simulink model "irep_force_control_simu"  (Simulink 8.5)
settings: Solver=ode3  StartTime=0.0  StopTime=inf  FixedStep=dt  RelTol=1e-3
InitFcn:
  | IREP_DEPENDENCY
  | init_omni
  | init_filters
  | init_invivo
  | init_telemanipulation
  | init_parker_xyz
  | init_magnetic_tracker
  | init_loadcell
  | init_scopes
  | init_homing
  | init_force_control
  | init_xpc_invivo_simu
undefined symbols (not defined in the file): ang_vel_scale, B_simu, beta, camera_home_voltage, counter_offset, dt, dt_trakstar, E_Y, encoder_counts, epsilon_robust_inverse, gear_ratio, HomingFineEps, HomingRoughEps, HomingRoughVelocity, I1_primary, I1_secondary, I2_primary, I2_secondary, irep_parameters_left, irep_parameters_right, joystick_filter_coeffs, K_d, K_i, K_naive_inv, K_p, k_right, L1l, L1r, L2l, L2r, L_zeus, left_arm_home_voltage, left_x0_parallelogram, LeftArmHomingDirectionVector, LeftArmHomingIntGain, lin_vel_scale, LOADCELL_BIAS, LOADCELL_GAIN, max_conf_space_speed, N_joystick, N_pots, N_trakstar, OmegaMax, OmegaMin, orientation_epsilon, position_epsilon, pots_filter_coeffs, q_eps_backlash, quadrature_mode, r, right_arm_home_voltage, RightArmHomingDirectionVector, RightArmHomingIntGain, screw_pitch, statics_param, tau_compression_bias, tau_compression_gains, tau_neutral_deadband, tau_tension_bias, tau_tension_gains ... (+14)
libraries: slrtlib x38, xpcrtudplib x13, xpcobsoletelib x13, simulink x6, dspswit3 x2, dspsigops x1
(part 1 of 6)
settings Model: Creator=Andrea  LastModifiedBy=Long
settings SolverCC: EnableConcurrentExecution=on
settings OptimizationCC: BlockReduction=off  OptimizeBlockIOStorage=off  BufferReuse=off  GlobalBufferReuse=off  ExpressionFolding=off  LocalBlockOutputs=off  OptimizeModelRefInitCode=on
settings DebuggingCC: SolverPrmCheckMsg=warning  MultiTaskCondExecSysMsg=warning  MultiTaskRateTransMsg=warning  FcnCallInpInsideContextMsg=UseLocalSettings
settings HardwareCC: ProdIntDivRoundTo=Zero  ProdEndianess=LittleEndian  ProdLongLongMode=on  ProdHWDeviceType=Generic->32-bit x86 compatible
settings SFSimCC: SimParseCustomCode=off
settings RTWCC: SystemTargetFile=slrtert.tlc  TemplateMakefile=slrtert_default_tmf  Description=Simulink Real-Time (ERT)  RTWCompilerOptimization=on
settings CodeAppCC: CustomSymbolStrType=$N$R$M  InternalIdentifier=Classic
settings SimulinkRealTimeERTCC: TargetFcnLib=ansi_tfl_table_tmw.mat  GenFloatMathFcnCalls=NOT IN USE  TargetLangStandard=C89/C90 (ANSI)  CodeReplacementLibrary=XPC_BLAS  UtilityFuncGeneration=Auto  ERTMultiwordTypeDef=System defined  ERTMultiwordLength=256  MultiwordLength=2048  GenerateFullHeader=on  InferredTypesCompatibility=off  GenerateSampleERTMain=off  GenerateTestInterfaces=off  ModelReferenceCompliant=on  ParMdlRefBuildCompliant=on  CompOptLevelCompliant=on  ConcurrentExecutionCompliant=on  IncludeMdlTerminateFcn=on  GeneratePreprocessorConditionals=Disable all  CombineOutputUpdateFcns=off  CombineSignalStateStructs=off  SuppressErrorStatus=off  ERTFirstTimeCompliant=off  IncludeFileDelimiter=Auto  ERTCustomFileBanners=off  SupportAbsoluteTime=on  LogVarNameModifier=rt_  MatFileLogging=on  MultiInstanceERTCode=off  CodeInterfacePackaging=Nonreusable function  SupportNonFinite=on  SupportComplex=on  PurelyIntegerCode=off  SupportContinuousTime=on  SupportNonInlinedSFcns=on  SupportVariableSizeSignals=off  ParenthesesLevel=Nominal  CastingMode=Nominal  MATLABClassNameForMDSCustomization=xpcAperiodicCustomization  ModelStepFunctionPrototypeControlCompliant=off  CPPClassGenCompliant=off  AutosarCompliant=off  GRTInterface=on  GenerateAllocFcn=off  GenerateSharedConstants=on  GenerateASAP2=off  ExtModeTransport=0  ExtModeStaticAlloc=off  ExtModeStaticAllocSize=1000000  ExtModeTesting=off  InlinedParameterPlacement=NonHierarchical  TargetOS=BareBoardExample  MultiInstanceErrorCode=Error  RateGroupingCode=on  RootIOFormat=Individual arguments  RTWCAPIRootIO=off  EnableDataOwnership=off  ERTFilePackagingFormat=Modular  PreserveExpressionOrder=off  PreserveIfCondition=off  ConvertIfToSwitch=off  PreserveExternInFcnDecls=on  SuppressUnreachableDefaultCases=off  EnableSignedLeftShifts=on  IndentStyle=K&R  IndentSize=2  EnableUserReplacementTypes=off  MaxIdInt32=MAX_int32_T  MinIdInt32=MIN_int32_T  MaxIdUint32=MAX_uint32_T  MaxIdInt16=MAX_int16_T  MinIdInt16=MIN_int16_T  MaxIdUint16=MAX_uint16_T  MaxIdInt8=MAX_int8_T  MinIdInt8=MIN_int8_T  MaxIdUint8=MAX_uint8_T  BooleanTrueId=true  BooleanFalseId=false  MemSecPackage=--- None ---  MemSecDataConstants=Default  MemSecDataIO=Default  MemSecDataInternal=Default  MemSecDataParameters=Default  MemSecFuncInitTerm=Default  MemSecFuncExecute=Default  MemSecFuncSharedUtil=Default  GlobalDataDefinition=Auto  GlobalDataReference=Auto  ERTSrcFileBannerTemplate=ert_code_template.cgt  ERTHdrFileBannerTemplate=ert_code_template.cgt  ERTDataSrcFileTemplate=ert_code_template.cgt  ERTDataHdrFileTemplate=ert_code_template.cgt  ERTCustomFileTemplate=example_file_process.tlc  SignalDisplayLevel=10  ParamTuneLevel=10  InitialValueSource=Model  RTWCAPISignals=off  RTWCAPIParams=on  RTWCAPIStates=off  RL32ModeModifier=Real-Time  ExtMode=on  ExtModeMexFile=ext_xpc  ExtModeIntrfLevel=Level2 - Open  ExtModeArmWhenConnect=off  RL32LogTETModifier=on  RL32LogBufSizeModifier=100000  xPCTaskExecutionProfile=off  xPCRL32EventNumber=5000  RL32IRQSourceModifier=Timer  xPCIRQSourceBoard=None/Other  xPCIOIRQSlot=-1  xpcObjCom=off  xPCGenerateASAP2=off  xPCGenerateXML=off  RL32ObjectName=tg  xPCisDownloadable=off  xPCisDefaultEnv=on  xPCisModelTimeout=on  xPCModelTimeoutSecs=5  xpcDblBuff=off  xPCLoadParamSetFile=off  xPCConcurrentTasks=off  xPCEnableSFAnimation=off

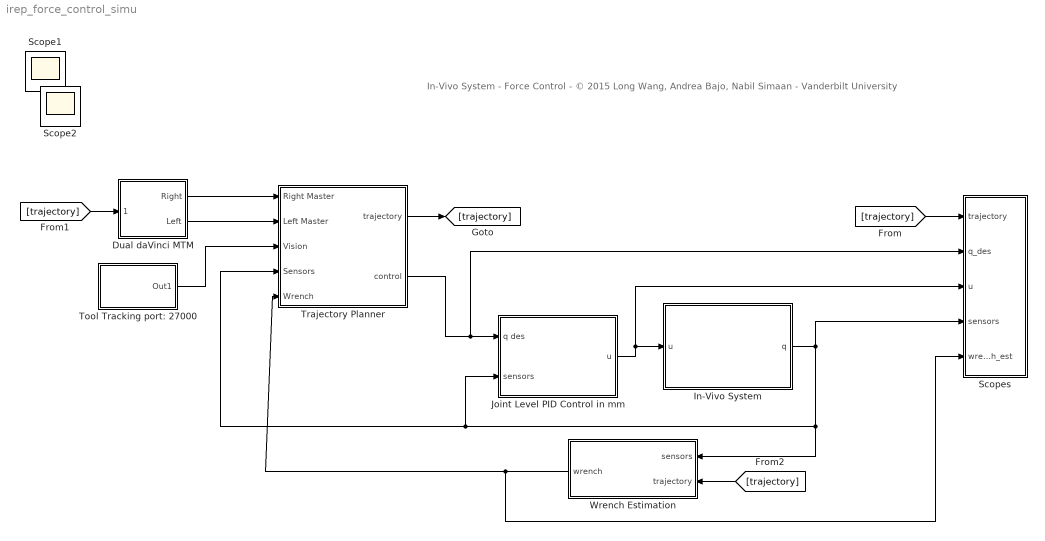
== system irep_force_control_simu ==
  note: In-Vivo System - Force Control - © 2015 Long Wang, Andrea Bajo, Nabil Simaan - Vanderbilt University
  Dual daVinci MTM : Subsystem
      mask Display: image(imread('davinci_doc.jpg'));
  In-Vivo System : Subsystem
      mask Display: image(imread('irep.png'));
  Joint Level PID Control in mm : Subsystem
  Scopes : Subsystem
  Tool Tracking port: 27000 : Subsystem  TreatAsAtomicUnit=on
  Trajectory Planner : Subsystem
  Wrench Estimation : Subsystem
  Scope1 : Scope
      settings: MaxDataPoints=7500
  Scope2 : Scope
      settings: MaxDataPoints=7500
  wires:
  In-Vivo System/1(q) -> Scopes/4(sensors), Trajectory Planner/4(Sensors), Joint Level PID Control in mm/2(sensors), Wrench Estimation/1(sensors)
  Trajectory Planner/2(control) -> Joint Level PID Control in mm/1(q des), Scopes/2(q_des)
  Tool Tracking port: 27000/1(Out1) -> Trajectory Planner/3(Vision)
  Dual daVinci MTM/2(Left) -> Trajectory Planner/2(Left Master)
  Dual daVinci MTM/1(Right) -> Trajectory Planner/1(Right Master)
  Wrench Estimation/1(wrench) -> Scopes/5(wrench_est), Trajectory Planner/5(Wrench)
  Trajectory Planner/1(trajectory) -> [trajectory]
  [trajectory] -> Scopes/1(trajectory)
  [trajectory] -> Dual daVinci MTM/1(trajectory)
  [trajectory] -> Wrench Estimation/2(trajectory)
  Joint Level PID Control in mm/1(u) -> Scopes/3(u), In-Vivo System/1(u)

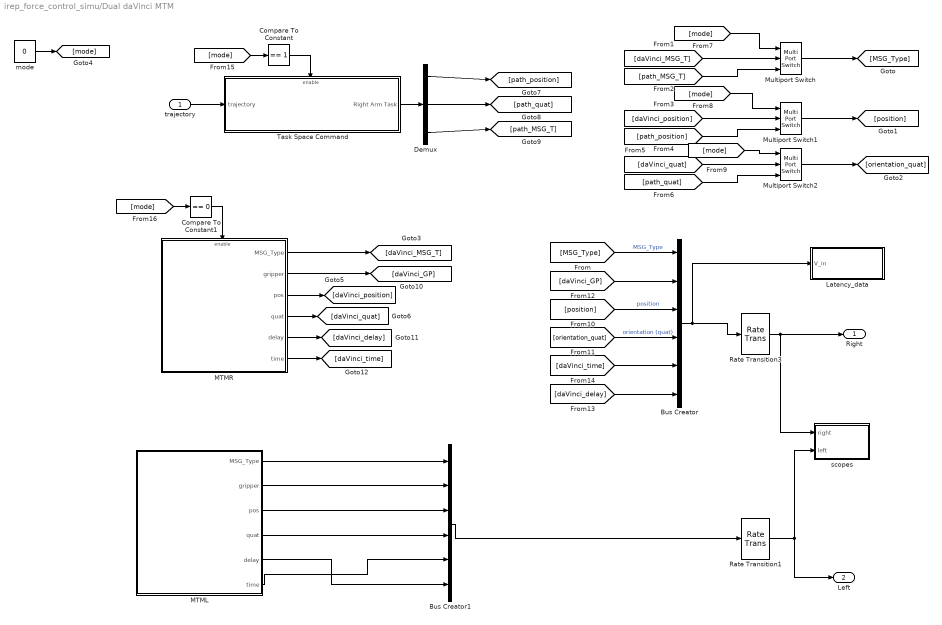
== system irep_force_control_simu/Dual daVinci MTM ==
  trajectory : Inport
  Bus Creator : BusCreator  Inputs=6
  Bus Creator1 : BusCreator  Inputs=6
  Compare To Constant : simulink/Logic and Bit Operations/Compare To Constant  relop===  const=1  OutDataTypeStr=boolean
  Compare To Constant1 : simulink/Logic and Bit Operations/Compare To Constant  relop===  const=0  OutDataTypeStr=boolean
  Demux : Demux  Outputs=[3,4,1]
  Latency_data : Subsystem
  MTML : Subsystem
  MTMR : Subsystem
  Multiport Switch : MultiPortSwitch  DataPortOrder=Zero-based contiguous  Inputs=2  zeroidx=on
  Multiport Switch1 : MultiPortSwitch  DataPortOrder=Zero-based contiguous  Inputs=2  zeroidx=on
  Multiport Switch2 : MultiPortSwitch  DataPortOrder=Zero-based contiguous  Inputs=2  zeroidx=on
  Rate Transition1 : RateTransition  OutPortSampleTime=dt
  Rate Transition3 : RateTransition  OutPortSampleTime=dt
  Task Space Command : Subsystem  TreatAsAtomicUnit=on
  mode : Constant  Value=0
  scopes : Subsystem
  Right : Outport
  Left : Outport  Port=2
  wires:
  Bus Creator/1 -> Latency_data/1(V_in), Rate Transition3/1
  Bus Creator1/1 -> Rate Transition1/1
  Rate Transition3/1 -> Right/1, scopes/1(right)
  Rate Transition1/1 -> Left/1, scopes/2(left)
  Multiport Switch/1 -> [MSG_Type]
  [MSG_Type] -> Bus Creator/1  "MSG_Type"
  Multiport Switch1/1 -> [position]
  Multiport Switch2/1 -> [orientation_quat]
  [daVinci_MSG_T] -> Multiport Switch/2
  [path_MSG_T] -> Multiport Switch/3
  [daVinci_position] -> Multiport Switch1/2
  [path_position] -> Multiport Switch1/3
  [daVinci_quat] -> Multiport Switch2/2
  [path_quat] -> Multiport Switch2/3
  mode/1 -> [mode]
  [mode] -> Multiport Switch/1
  [mode] -> Multiport Switch1/1
  [mode] -> Multiport Switch2/1
  [position] -> Bus Creator/3  "position"
  [orientation_quat] -> Bus Creator/4  "orientation (quat)"
  trajectory/1 -> Task Space Command/1(trajectory)
  Task Space Command/1(Right Arm Task) -> Demux/1
  MTMR/4(quat) -> [daVinci_quat]
  MTMR/3(pos) -> [daVinci_position]
  MTMR/1(MSG_Type) -> [daVinci_MSG_T]
  MTMR/2(gripper) -> [daVinci_GP]
  [daVinci_GP] -> Bus Creator/2
  MTMR/5(delay) -> [daVinci_delay]
  [daVinci_delay] -> Bus Creator/6
  MTMR/6(time) -> [daVinci_time]
  [daVinci_time] -> Bus Creator/5
  [mode] -> Compare To Constant/1
  Compare To Constant/1 -> Task Space Command/Enable
  [mode] -> Compare To Constant1/1
  Compare To Constant1/1 -> MTMR/Enable
  MTML/1(MSG_Type) -> Bus Creator1/1
  MTML/2(gripper) -> Bus Creator1/2
  MTML/3(pos) -> Bus Creator1/3
  MTML/4(quat) -> Bus Creator1/4
  MTML/6(time) -> Bus Creator1/5
  MTML/5(delay) -> Bus Creator1/6
  Demux/1 -> [path_position]
  Demux/2 -> [path_quat]
  Demux/3 -> [path_MSG_T]

== system irep_force_control_simu/In-Vivo System ==
  u : Inport
  ATI FT Sensor : Subsystem
  Bus Creator : BusCreator  Inputs=7
  CONTEC CARDS : Subsystem
  Count to mm : Subsystem
  D/A : Subsystem
  Digital_Inputs : Subsystem
  Loadcells : Subsystem
  Magnetic Tracker 125 Hz : Subsystem  TreatAsAtomicUnit=on
      mask Display: %image(imread('trakSTAR.jpg'));
  Motor Enable : Subsystem
  Potentiometers : Subsystem
  Terminator : Terminator
  motor simulation : Subsystem
  q : Outport
  wires:
  CONTEC CARDS/1(Out1) -> Count to mm/1(counts)
  u/1 -> D/A/1(In1), motor simulation/1(u)
  Potentiometers/1(Pots) -> Bus Creator/2  "A/D signals"
  Bus Creator/1 -> q/1
  Digital_Inputs/1(foot switches) -> Bus Creator/3  "foot switches"
  Digital_Inputs/2(Pot_connect) -> Bus Creator/4  "Pots_Connect"
  ATI FT Sensor/1(Forces) -> Bus Creator/6  "ATI"
  Loadcells/1(loadcell) -> Bus Creator/7  "force_sensing"
  Magnetic Tracker 125 Hz/1(TrakStar) -> Bus Creator/5  "Magnetic Sensors"
  motor simulation/1(q_cur_system) -> Bus Creator/1  "q"
  Count to mm/1(q_cur_system) -> Terminator/1  "q"

== system irep_force_control_simu/Joint Level PID Control in mm ==
  q des : Inport
  sensors : Inport  Port=2
  Bus Creator : Subsystem
  Bus selector : Subsystem
  Enable Control : Constant  Value=0
  PID Compensator : Subsystem
  Sum : Sum  Inputs=|+-  SampleTime=dt
  u : Outport
  wires:
  q des/1 -> Sum/1
  Sum/1 -> PID Compensator/1(e)
  sensors/1 -> Bus selector/1(sensors)
  Bus selector/1(Out1) -> Sum/2
  PID Compensator/1(u) -> Bus Creator/1(In1)
  Bus Creator/1(Out1) -> u/1
  Enable Control/1 -> PID Compensator/Enable

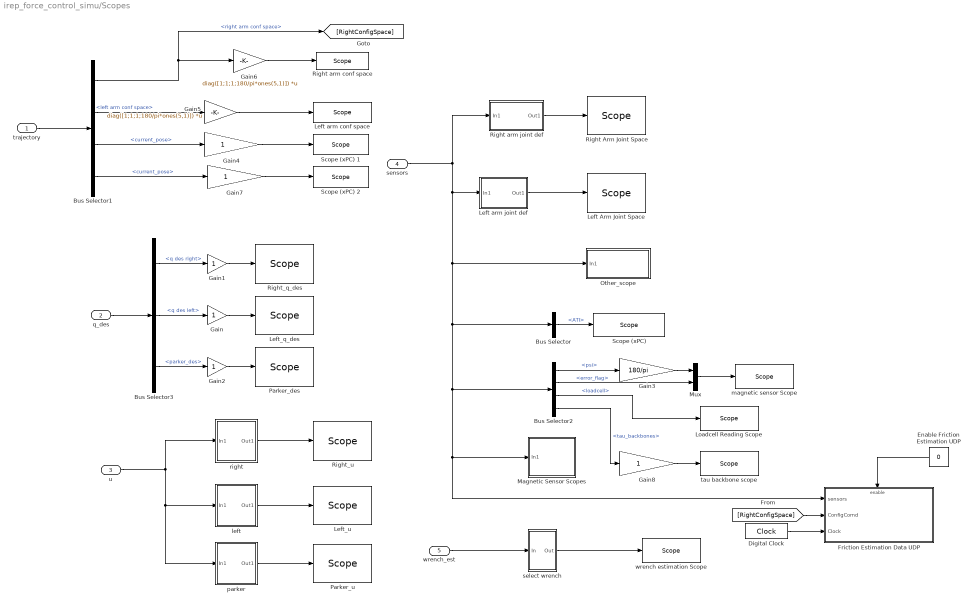
== system irep_force_control_simu/Scopes ==
  trajectory : Inport
  q_des : Inport  Port=2
  u : Inport  Port=3
  sensors : Inport  Port=4
  wrench_est : Inport  Port=5
  Bus Selector : BusSelector  OutputSignals=ATI
  Bus Selector1 : BusSelector  OutputSignals=right arm.right arm conf space,left arm.left arm conf space,right arm.current_pose,left arm.current_pose
  Bus Selector2 : BusSelector  OutputSignals=Magnetic Sensors.psi,Magnetic Sensors.error_flag,force_sensing.loadcell,force_sensing.tau_backbones
  Bus Selector3 : BusSelector  OutputSignals=q des right,q des left,parker_des
  Digital Clock : DigitalClock  SampleTime=dt
  Enable Friction Estimation UDP : Constant  Value=0
  Friction Estimation Data UDP : Subsystem
  Gain{,1..2,4,7..8} (6 alike) : Gain
  Gain3 : Gain  Gain=180/pi
  Gain5 : Gain  Gain=diag([1;1;1;180/pi*ones(5,1)])  Multiplication=Matrix(K*u)
  Gain6 : Gain  Gain=diag([1;1;1;180/pi*ones(5,1)])  Multiplication=Matrix(K*u)
  Left Arm Joint Space : slrtlib/Displays and Logging/Scope   scopeno=5  scopetype=Host  autostart=on  viewmode=Numerical  formatstr=scope_format_left_joint_space  grid=on  ylimits=[0,0]  nosamples=10  noprepostsamples=0  interleave=1  triggermode=FreeRun  triggersignal=1  trigsignalfromport=off  triggerlevel=0.0  triggerslope=Either  triggerscope=1  triggersample=0  filename=weights1.dat  mode=Lazy  writesize=512  autorestart=off  dynamicfilemode=off  maxwritefilesize=512*1024^2
  Left arm conf space : slrtlib/Displays and Logging/Scope   scopeno=10  scopetype=Target  autostart=on  viewmode=Numerical  formatstr=scope_format_left_config_space  grid=on  ylimits=[0,0]  nosamples=10  noprepostsamples=0  interleave=1  triggermode=FreeRun  triggersignal=1  trigsignalfromport=off  triggerlevel=0.0  triggerslope=Either  triggerscope=1  triggersample=0  filename=weights.dat  mode=Lazy  writesize=512  autorestart=off  dynamicfilemode=off  maxwritefilesize=512*1024^2
  Left arm joint def : Subsystem
  Left_q_des : slrtlib/Displays and Logging/Scope   scopeno=13  scopetype=Target  autostart=on  viewmode=Numerical  formatstr=scope_format_left_q_des  grid=on  ylimits=[0,0]  nosamples=10  noprepostsamples=0  interleave=1  triggermode=FreeRun  triggersignal=1  trigsignalfromport=off  triggerlevel=0.0  triggerslope=Either  triggerscope=1  triggersample=0  filename=weights.dat  mode=Lazy  writesize=512  autorestart=off  dynamicfilemode=off  maxwritefilesize=512*1024^2
  Left_u : slrtlib/Displays and Logging/Scope   scopeno=15  scopetype=Host  autostart=on  viewmode=Numerical  formatstr=scope_format_left_u  grid=on  ylimits=[0,0]  nosamples=10  noprepostsamples=0  interleave=1  triggermode=FreeRun  triggersignal=1  trigsignalfromport=off  triggerlevel=0.0  triggerslope=Either  triggerscope=1  triggersample=0  filename=weights.dat  mode=Lazy  writesize=512  autorestart=off  dynamicfilemode=off  maxwritefilesize=512*1024^2
  Loadcell Reading Scope : slrtlib/Displays and Logging/Scope   scopeno=29  scopetype=Host  autostart=on  viewmode=Numerical  formatstr=scope_format_Loadcell  grid=on  ylimits=[0,0]  nosamples=25  noprepostsamples=0  interleave=1  triggermode=FreeRun  triggersignal=1  trigsignalfromport=off  triggerlevel=0.0  triggerslope=Either  triggerscope=1  triggersample=0  filename=data.dat  mode=Lazy  writesize=512  autorestart=off  dynamicfilemode=off  maxwritefilesize=512*1024^2
  Magnetic Sensor Scopes : Subsystem
  Mux : Mux  Inputs=2
  Other_scope : Subsystem
  Parker_des : slrtlib/Displays and Logging/Scope   scopeno=17  scopetype=Host  autostart=on  viewmode=Numerical  formatstr=scope_format_parker_des  grid=on  ylimits=[0,0]  nosamples=10  noprepostsamples=0  interleave=1  triggermode=FreeRun  triggersignal=1  trigsignalfromport=off  triggerlevel=0.0  triggerslope=Either  triggerscope=1  triggersample=0  filename=weights.dat  mode=Lazy  writesize=512  autorestart=off  dynamicfilemode=off  maxwritefilesize=512*1024^2
  Parker_u : slrtlib/Displays and Logging/Scope   scopeno=16  scopetype=Host  autostart=on  viewmode=Numerical  formatstr=scope_format_parker_u  grid=on  ylimits=[0,0]  nosamples=10  noprepostsamples=0  interleave=1  triggermode=FreeRun  triggersignal=1  trigsignalfromport=off  triggerlevel=0.0  triggerslope=Either  triggerscope=1  triggersample=0  filename=weights.dat  mode=Lazy  writesize=512  autorestart=off  dynamicfilemode=off  maxwritefilesize=512*1024^2
  Right Arm Joint Space : slrtlib/Displays and Logging/Scope   scopeno=3  scopetype=Host  autostart=on  viewmode=Numerical  formatstr=scope_format_right_joint_space  grid=on  ylimits=[0,0]  nosamples=10  noprepostsamples=0  interleave=1  triggermode=FreeRun  triggersignal=1  trigsignalfromport=off  triggerlevel=0.0  triggerslope=Either  triggerscope=1  triggersample=0  filename=weights1.dat  mode=Lazy  writesize=512  autorestart=off  dynamicfilemode=off  maxwritefilesize=512*1024^2
  Right arm conf space : slrtlib/Displays and Logging/Scope   scopeno=9  scopetype=Host  autostart=on  viewmode=Numerical  formatstr=scope_format_right_config_space  grid=on  ylimits=[0,0]  nosamples=10  noprepostsamples=0  interleave=1  triggermode=FreeRun  triggersignal=1  trigsignalfromport=off  triggerlevel=0.0  triggerslope=Either  triggerscope=1  triggersample=0  filename=weights.dat  mode=Lazy  writesize=512  autorestart=off  dynamicfilemode=off  maxwritefilesize=512*1024^2
  Right arm joint def : Subsystem
  Right_q_des : slrtlib/Displays and Logging/Scope   scopeno=12  scopetype=Host  autostart=on  viewmode=Numerical  formatstr=scope_format_right_q_des  grid=on  ylimits=[0,0]  nosamples=10  noprepostsamples=0  interleave=1  triggermode=FreeRun  triggersignal=1  trigsignalfromport=off  triggerlevel=0.0  triggerslope=Either  triggerscope=1  triggersample=0  filename=weights.dat  mode=Lazy  writesize=512  autorestart=off  dynamicfilemode=off  maxwritefilesize=512*1024^2
  Right_u : slrtlib/Displays and Logging/Scope   scopeno=14  scopetype=Host  autostart=on  viewmode=Numerical  formatstr=scope_format_right_config_space  grid=on  ylimits=[0,0]  nosamples=10  noprepostsamples=0  interleave=1  triggermode=FreeRun  triggersignal=1  trigsignalfromport=off  triggerlevel=0.0  triggerslope=Either  triggerscope=1  triggersample=0  filename=weights.dat  mode=Lazy  writesize=512  autorestart=off  dynamicfilemode=off  maxwritefilesize=512*1024^2
  "Scope (xPC) " : slrtlib/Displays and Logging/Scope   scopeno=20  scopetype=Host  autostart=on  viewmode=Numerical  formatstr=scope_format_ATI_wrench  grid=on  ylimits=[0,0]  nosamples=25  noprepostsamples=0  interleave=1  triggermode=FreeRun  triggersignal=1  trigsignalfromport=off  triggerlevel=0.0  triggerslope=Either  triggerscope=1  triggersample=0  filename=data.dat  mode=Lazy  writesize=512  autorestart=off  dynamicfilemode=off  maxwritefilesize=512*1024^2
  Scope (xPC) 1 : slrtlib/Displays and Logging/Scope   scopeno=36  scopetype=Host  autostart=on  viewmode=Numerical  formatstr=scope_format_right_task_space_cur  grid=on  ylimits=[0,0]  nosamples=25  noprepostsamples=0  interleave=1  triggermode=FreeRun  triggersignal=1  trigsignalfromport=off  triggerlevel=0.0  triggerslope=Either  triggerscope=1  triggersample=0  filename=data.dat  mode=Lazy  writesize=512  autorestart=off  dynamicfilemode=off  maxwritefilesize=512*1024^2
  Scope (xPC) 2 : slrtlib/Displays and Logging/Scope   scopeno=37  scopetype=Host  autostart=on  viewmode=Numerical  formatstr=scope_format_left_task_space_cur  grid=on  ylimits=[0,0]  nosamples=25  noprepostsamples=0  interleave=1  triggermode=FreeRun  triggersignal=1  trigsignalfromport=off  triggerlevel=0.0  triggerslope=Either  triggerscope=1  triggersample=0  filename=data.dat  mode=Lazy  writesize=512  autorestart=off  dynamicfilemode=off  maxwritefilesize=512*1024^2
  left : Subsystem
  magnetic sensor Scope : slrtlib/Displays and Logging/Scope   scopeno=33  scopetype=Host  autostart=on  viewmode=Numerical  formatstr=scope_format_megnetic_psi  grid=on  ylimits=[0,0]  nosamples=25  noprepostsamples=0  interleave=1  triggermode=FreeRun  triggersignal=1  trigsignalfromport=off  triggerlevel=0.0  triggerslope=Either  triggerscope=1  triggersample=0  filename=data.dat  mode=Lazy  writesize=512  autorestart=off  dynamicfilemode=off  maxwritefilesize=512*1024^2
  parker : Subsystem
  right : Subsystem
  select wrench : Subsystem
  tau backbone scope : slrtlib/Displays and Logging/Scope   scopeno=34  scopetype=Host  autostart=on  viewmode=Numerical  formatstr=scope_format_tau_backbones  grid=on  ylimits=[0,0]  nosamples=50  noprepostsamples=0  interleave=1  triggermode=FreeRun  triggersignal=1  trigsignalfromport=off  triggerlevel=0.0  triggerslope=Either  triggerscope=1  triggersample=0  filename=data.dat  mode=Lazy  writesize=512  autorestart=off  dynamicfilemode=off  maxwritefilesize=512*1024^2
  wrench estimation Scope : slrtlib/Displays and Logging/Scope   scopeno=35  scopetype=Host  autostart=on  viewmode=Numerical  formatstr=scope_format_wrench_est_right_arm  grid=on  ylimits=[0,0]  nosamples=25  noprepostsamples=0  interleave=1  triggermode=FreeRun  triggersignal=1  trigsignalfromport=off  triggerlevel=0.0  triggerslope=Either  triggerscope=1  triggersample=0  filename=data.dat  mode=Lazy  writesize=512  autorestart=off  dynamicfilemode=off  maxwritefilesize=512*1024^2
  wires:
  sensors/1 -> Other_scope/1(In1), Bus Selector/1, Bus Selector2/1, Magnetic Sensor Scopes/1(In1), Friction Estimation Data UDP/1(sensors), Left arm joint def/1(In1), Right arm joint def/1(In1)
  trajectory/1 -> Bus Selector1/1
  Bus Selector1/1 -> [RightConfigSpace], Gain6/1  "<right arm conf space>"
  Bus Selector1/2 -> Gain5/1  "<left arm conf space>"
  q_des/1 -> Bus Selector3/1
  Bus Selector3/1 -> Gain1/1  "<q des right>"
  Bus Selector3/2 -> Gain/1  "<q des left>"
  u/1 -> right/1(In1), left/1(In1), parker/1(In1)
  right/1(Out1) -> Right_u/1
  left/1(Out1) -> Left_u/1
  Gain/1 -> Left_q_des/1
  Gain1/1 -> Right_q_des/1
  parker/1(Out1) -> Parker_u/1
  Bus Selector3/3 -> Gain2/1  "<parker_des>"
  Gain2/1 -> Parker_des/1
  Right arm joint def/1(Out1) -> Right Arm Joint Space/1
  Left arm joint def/1(Out1) -> Left Arm Joint Space/1
  Bus Selector/1 -> "Scope (xPC) "/1  "<ATI>"
  Bus Selector2/1 -> Gain3/1  "<psi>"
  [RightConfigSpace] -> Friction Estimation Data UDP/2(ConfigComd)
  Enable Friction Estimation UDP/1 -> Friction Estimation Data UDP/Enable
  Digital Clock/1 -> Friction Estimation Data UDP/3(Clock)
  Bus Selector2/3 -> Loadcell Reading Scope/1  "<loadcell>"
  Bus Selector2/4 -> Gain8/1  "<tau_backbones>"
  wrench_est/1 -> select wrench/1(In)
  select wrench/1(Out) -> wrench estimation Scope/1
  Bus Selector2/2 -> Mux/2  "<error_flag>"
  Gain3/1 -> Mux/1
  Mux/1 -> magnetic sensor Scope/1
  Gain4/1 -> Scope (xPC) 1/1
  Gain5/1 -> Left arm conf space/1
  Gain6/1 -> Right arm conf space/1
  Gain7/1 -> Scope (xPC) 2/1
  Bus Selector1/4 -> Gain7/1  "<current_pose>"
  Bus Selector1/3 -> Gain4/1  "<current_pose>"
  Gain8/1 -> tau backbone scope/1

== system irep_force_control_simu/Tool Tracking port: 27000 ==
  Camera : slrtlib/Displays and Logging/Scope   scopeno=1  scopetype=Host  autostart=on  viewmode=Numerical  formatstr='Pixels: %3.2f'  grid=on  ylimits=[0,0]  nosamples=10  noprepostsamples=0  interleave=1  triggermode=FreeRun  triggersignal=1  trigsignalfromport=off  triggerlevel=0.0  triggerslope=Either  triggerscope=1  triggersample=0  filename=weights1.dat  mode=Lazy  writesize=512  autorestart=off  dynamicfilemode=off  maxwritefilesize=512*1024^2
  Mux : Mux
  Rate Transition3 : RateTransition  OutPortSampleTime=dt
  Receive : xpcrtudplib/Legacy UDP/Receive   ipAddress=0.0.0.0  ipPort=27000  width=32  vblLen=on  sampletime=dt_omni
  Terminator : Terminator
  Unpack : xpcobsoletelib/Utilities/Unpack   dimensions={1,1,1,1}  datatypes={'double' 'double' 'double' 'double'}  byteAlign=1
  compute offset : MATLAB Function  TreatAsAtomicUnit=on
  Out1 : Outport
  wires:
  Receive/2 -> Terminator/1
  Receive/1 -> Unpack/1
  Unpack/1 -> Mux/1
  Unpack/2 -> Mux/2
  Mux/1 -> compute offset/1(u)
  compute offset/1(y) -> Rate Transition3/1, Camera/1
  Unpack/3 -> Mux/3
  Unpack/4 -> Mux/4
  Rate Transition3/1 -> Out1/1

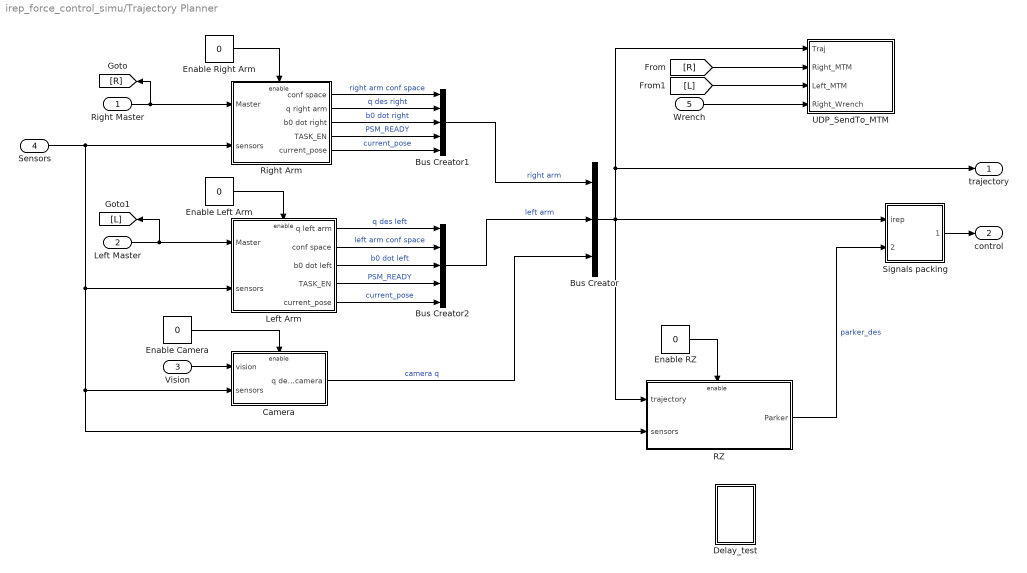
== system irep_force_control_simu/Trajectory Planner ==
  Right Master : Inport
  Left Master : Inport  Port=2
  Vision : Inport  Port=3
  Sensors : Inport  Port=4
  Wrench : Inport  Port=5
  Bus Creator : BusCreator  Inputs=3
  Bus Creator1 : BusCreator  Inputs=5
  Bus Creator2 : BusCreator  Inputs=5
  Camera : Subsystem  TreatAsAtomicUnit=on
  Delay_test : Subsystem
  Enable Camera : Constant  Value=0  SampleTime=dt
  Enable Left Arm : Constant  Value=0  SampleTime=dt
  Enable RZ : Constant  Value=0  SampleTime=dt
  Enable Right Arm : Constant  Value=0  SampleTime=dt
  Left Arm : Subsystem  TreatAsAtomicUnit=on
  RZ : Subsystem  TreatAsAtomicUnit=on
  Right Arm : Subsystem  TreatAsAtomicUnit=on
  Signals packing : Subsystem
  UDP_SendTo_MTM : Subsystem
  trajectory : Outport  SampleTime=dt
  control : Outport  Port=2  PortDimensions=[23 1]  SampleTime=dt
  wires:
  Enable Right Arm/1 -> Right Arm/Enable
  Enable Left Arm/1 -> Left Arm/Enable
  Enable Camera/1 -> Camera/Enable
  Right Master/1 -> Right Arm/1(Master), [R]
  Signals packing/1(system) -> control/1
  Sensors/1 -> Left Arm/2(sensors), Camera/2(sensors), RZ/2(sensors), Right Arm/2(sensors)
  Vision/1 -> Camera/1(vision)
  Left Master/1 -> Left Arm/1(Master), [L]
  Enable RZ/1 -> RZ/Enable
  Right Arm/2(q right arm) -> Bus Creator1/2  "q des right"
  Right Arm/1(conf space) -> Bus Creator1/1  "right arm conf space"
  Right Arm/3(b0 dot right) -> Bus Creator1/3  "b0 dot right"
  Left Arm/2(conf space) -> Bus Creator2/2  "left arm conf space"
  Left Arm/1(q left arm) -> Bus Creator2/1  "q des left"
  Bus Creator1/1 -> Bus Creator/1  "right arm"
  Bus Creator2/1 -> Bus Creator/2  "left arm"
  Camera/1(q des camera) -> Bus Creator/3  "camera q"
  Bus Creator/1 -> RZ/1(trajectory), Signals packing/1(irep), trajectory/1, UDP_SendTo_MTM/1(Traj)
  RZ/1(Parker) -> Signals packing/2(parker)  "parker_des"
  Left Arm/3(b0 dot left) -> Bus Creator2/3  "b0 dot left"
  Right Arm/4(TASK_EN) -> Bus Creator1/4  "PSM_READY"
  Left Arm/4(TASK_EN) -> Bus Creator2/4  "PSM_READY"
  [R] -> UDP_SendTo_MTM/2(Right_MTM)
  [L] -> UDP_SendTo_MTM/3(Left_MTM)
  Right Arm/5(current_pose) -> Bus Creator1/5  "current_pose"
  Wrench/1 -> UDP_SendTo_MTM/4(Right_Wrench)
  Left Arm/5(current_pose) -> Bus Creator2/5  "current_pose"

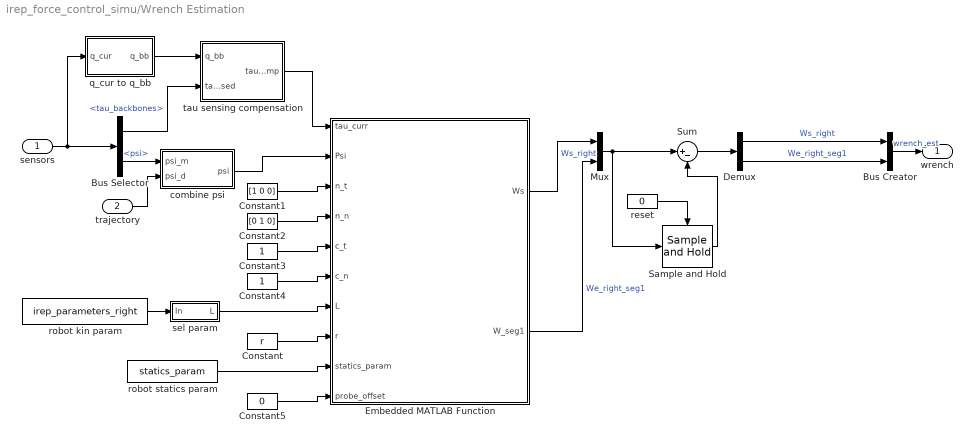
== system irep_force_control_simu/Wrench Estimation ==
  sensors : Inport
  trajectory : Inport  Port=2
  Bus Creator : BusCreator  Inputs=2
  Bus Selector : BusSelector  OutputSignals=force_sensing.tau_backbones,Magnetic Sensors.psi
  Constant : Constant  Value=r
  Constant1 : Constant  Value=[1 0 0]
  Constant2 : Constant  Value=[0 1 0]
  Constant3 : Constant
  Constant4 : Constant
  Constant5 : Constant  Value=0
  Demux : Demux  Outputs=2
  Embedded MATLAB Function : MATLAB Function  TreatAsAtomicUnit=on
  Mux : Mux  Inputs=2
  Sample and Hold : dspsigops/Sample and Hold  trig=Rising edge  initCond=0  latchinput=off
  Sum : Sum  Inputs=|+-
  combine psi : Subsystem
  q_cur to q_bb : Subsystem
  reset : Constant  Value=0
  robot kin param : Constant  Value=irep_parameters_right
  robot statics param : Constant  Value=statics_param
  sel param : Subsystem
  tau sensing compensation : Subsystem
  wrench : Outport
  wires:
  Constant/1 -> Embedded MATLAB Function/8(r)
  Constant1/1 -> Embedded MATLAB Function/3(n_t)
  Constant2/1 -> Embedded MATLAB Function/4(n_n)
  Constant3/1 -> Embedded MATLAB Function/5(c_t)
  Constant4/1 -> Embedded MATLAB Function/6(c_n)
  robot kin param/1 -> sel param/1(In)
  sel param/1(L) -> Embedded MATLAB Function/7(L)
  robot statics param/1 -> Embedded MATLAB Function/9(statics_param)
  Constant5/1 -> Embedded MATLAB Function/10(probe_offset)
  sensors/1 -> Bus Selector/1, q_cur to q_bb/1(q_cur)
  Bus Selector/1 -> tau sensing compensation/2(tau_sensed)  "<tau_backbones>"
  reset/1 -> Sample and Hold/Trigger
  Bus Creator/1 -> wrench/1  "wrench_est"
  Embedded MATLAB Function/1(Ws) -> Mux/1  "Ws_right"
  Embedded MATLAB Function/2(W_seg1) -> Mux/2  "We_right_seg1"
  Mux/1 -> Sum/1, Sample and Hold/1
  Sample and Hold/1 -> Sum/2
  Sum/1 -> Demux/1
  Demux/1 -> Bus Creator/1  "Ws_right"
  Demux/2 -> Bus Creator/2  "We_right_seg1"
  q_cur to q_bb/1(q_bb) -> tau sensing compensation/1(q_bb)
  tau sensing compensation/1(tau_comp) -> Embedded MATLAB Function/1(tau_curr)
  Bus Selector/2 -> combine psi/1(psi_m)  "<psi>"
  trajectory/1 -> combine psi/2(psi_d)
  combine psi/1(psi) -> Embedded MATLAB Function/2(Psi)

== system irep_force_control_simu/Dual daVinci MTM/Latency_data ==
  V_in : Inport
  Discrete FIR Filter : DiscreteFir  CoefSource=Input port  AccumDataTypeStr=Inherit: Same as product output
  Gain : Gain  Gain=1/10
  Terminator : Terminator
  filter_coeffs : Constant  Value=ones(10,1)
  wires:
  V_in/1 -> Discrete FIR Filter/1
  Discrete FIR Filter/1 -> Gain/1
  filter_coeffs/1 -> Discrete FIR Filter/2
  Gain/1 -> Terminator/1

== system irep_force_control_simu/Dual daVinci MTM/MTML ==
  Embedded MATLAB Function : MATLAB Function  TreatAsAtomicUnit=on
  Embedded MATLAB Function1 : MATLAB Function  TreatAsAtomicUnit=on
  Mux1 : Mux  Inputs=3
  Mux5 : Mux  Inputs=9
  Receive : xpcrtudplib/Legacy UDP/Receive   ipAddress=0.0.0.0  ipPort=10004  width=8*22  vblLen=on  sampletime=dt_omni
  Terminator{,2..7} (7 alike) : Terminator
  Unpack : xpcobsoletelib/Utilities/Unpack   dimensions={1,1,1,1,1,1,1,1,1,1,1,1,1,1,1,1,1,1,1,1,1,1}  datatypes={'double' 'double' 'double' 'double' 'double' 'double' 'double' 'double' 'double' 'double' 'double' 'double' 'double' 'double' 'double' 'double' 'double' 'double' 'double' 'double' 'double' 'double'}  byteAlign=1
  m to mm : Gain  Gain=1000
  sec to msec : Gain  Gain=1000
  MSG_Type : Outport
  gripper : Outport  Port=2
  pos : Outport  Port=3
  quat : Outport  Port=4
  delay : Outport  Port=5
  time : Outport  Port=6
  wires:
  Unpack/21 -> time/1  "MTM_time"
  sec to msec/1 -> delay/1  "Delay"
  Embedded MATLAB Function1/1(quat) -> quat/1  "orientation (quat)"
  m to mm/1 -> pos/1  "position"
  Unpack/2 -> gripper/1  "gripper"
  Unpack/1 -> MSG_Type/1  "MSG_Type"
  Receive/2 -> Terminator/1
  Receive/1 -> Unpack/1
  Unpack/5 -> Mux1/3  "z"
  Unpack/4 -> Mux1/2  "y"
  Unpack/3 -> Mux1/1  "x"
  Mux1/1 -> m to mm/1
  Unpack/22 -> sec to msec/1
  Unpack/6 -> Mux5/1  "R11"
  Unpack/7 -> Mux5/2  "R21"
  Unpack/8 -> Mux5/3  "R31"
  Unpack/9 -> Mux5/4  "R12"
  Unpack/10 -> Mux5/5  "R22"
  Unpack/11 -> Mux5/6  "R32"
  Unpack/12 -> Mux5/7  "R13"
  Unpack/13 -> Mux5/8  "R23"
  Unpack/14 -> Mux5/9  "R33"
  Mux5/1 -> Embedded MATLAB Function/1(R_vec)
  Embedded MATLAB Function/1(R) -> Embedded MATLAB Function1/1(R)
  Unpack/15 -> Terminator5/1
  Unpack/16 -> Terminator2/1
  Unpack/17 -> Terminator3/1
  Unpack/18 -> Terminator4/1
  Unpack/20 -> Terminator7/1
  Unpack/19 -> Terminator6/1

== system irep_force_control_simu/Dual daVinci MTM/MTMR ==
  Enable : EnablePort  StatesWhenEnabling=reset
  Embedded MATLAB Function : MATLAB Function  TreatAsAtomicUnit=on
  Embedded MATLAB Function1 : MATLAB Function  TreatAsAtomicUnit=on
  Mux1 : Mux  Inputs=3
  Mux5 : Mux  Inputs=9
  Receive : xpcrtudplib/Legacy UDP/Receive   ipAddress=0.0.0.0  ipPort=10005  width=8*22  vblLen=on  sampletime=dt_omni
  Terminator{,2..7} (7 alike) : Terminator
  Unpack : xpcobsoletelib/Utilities/Unpack   dimensions={1,1,1,1,1,1,1,1,1,1,1,1,1,1,1,1,1,1,1,1,1,1}  datatypes={'double' 'double' 'double' 'double' 'double' 'double' 'double' 'double' 'double' 'double' 'double' 'double' 'double' 'double' 'double' 'double' 'double' 'double' 'double' 'double' 'double' 'double'}  byteAlign=1
  m to mm : Gain  Gain=1000
  sec to msec : Gain  Gain=1000
  MSG_Type : Outport
  gripper : Outport  Port=2
  pos : Outport  Port=3
  quat : Outport  Port=4
  delay : Outport  Port=5
  time : Outport  Port=6
  wires:
  Unpack/19 -> Terminator6/1
  Unpack/20 -> Terminator7/1
  Unpack/18 -> Terminator4/1
  Unpack/17 -> Terminator3/1
  Unpack/16 -> Terminator2/1
  Unpack/15 -> Terminator5/1
  Embedded MATLAB Function/1(R) -> Embedded MATLAB Function1/1(R)
  Mux5/1 -> Embedded MATLAB Function/1(R_vec)
  Unpack/14 -> Mux5/9  "R33"
  Unpack/13 -> Mux5/8  "R23"
  Unpack/12 -> Mux5/7  "R13"
  Unpack/11 -> Mux5/6  "R32"
  Unpack/10 -> Mux5/5  "R22"
  Unpack/9 -> Mux5/4  "R12"
  Unpack/8 -> Mux5/3  "R31"
  Unpack/7 -> Mux5/2  "R21"
  Unpack/6 -> Mux5/1  "R11"
  Unpack/22 -> sec to msec/1
  Mux1/1 -> m to mm/1
  Unpack/3 -> Mux1/1  "x"
  Unpack/4 -> Mux1/2  "y"
  Unpack/5 -> Mux1/3  "z"
  Receive/1 -> Unpack/1
  Receive/2 -> Terminator/1
  Unpack/1 -> MSG_Type/1  "MSG_Type"
  Unpack/2 -> gripper/1  "gripper"
  m to mm/1 -> pos/1  "position"
  Embedded MATLAB Function1/1(quat) -> quat/1  "orientation (quat)"
  sec to msec/1 -> delay/1  "Delay"
  Unpack/21 -> time/1  "MTM_time"

== system irep_force_control_simu/Dual daVinci MTM/Task Space Command ==
  trajectory : Inport
  Enable : EnablePort  StatesWhenEnabling=reset
  Bus Selector : BusSelector  OutputSignals=right arm.current_pose.p in world,left arm.current_pose.quat
  Mux : Mux  Inputs=[3,4,1]
  Right Arm - 5th Order Polynomial and Slerp : Subsystem
  Terminator : Terminator
  Unit Delay : UnitDelay  InitialCondition=zeros(3,1)  SampleTime=-1
  Unit Delay1 : UnitDelay  InitialCondition=[1;0;0;0]  SampleTime=-1
  go : Constant  Value=0
  p_ref : Constant  Value=[0;0;0]
  quat_ref : Constant  Value=[1;0;0;0]
  Right Arm Task : Outport  InitialOutput=zeros(8,1)
  wires:
  trajectory/1 -> Bus Selector/1
  p_ref/1 -> Right Arm - 5th Order Polynomial and Slerp/1(p_ref)
  Right Arm - 5th Order Polynomial and Slerp/2(quat_des) -> Mux/2  "Quat"
  quat_ref/1 -> Right Arm - 5th Order Polynomial and Slerp/2(quat_ref)
  go/1 -> Mux/3, Right Arm - 5th Order Polynomial and Slerp/5(enable)  "Enable"
  Right Arm - 5th Order Polynomial and Slerp/3(RecordFlag) -> Terminator/1  "InProcess"
  Bus Selector/1 -> Unit Delay/1  "<p in world>"
  Bus Selector/2 -> Unit Delay1/1  "<quat>"
  Right Arm - 5th Order Polynomial and Slerp/1(p_des) -> Mux/1  "position in mm"
  Mux/1 -> Right Arm Task/1
  Unit Delay/1 -> Right Arm - 5th Order Polynomial and Slerp/3(p curr)
  Unit Delay1/1 -> Right Arm - 5th Order Polynomial and Slerp/4(quat curr)

== system irep_force_control_simu/Dual daVinci MTM/scopes ==
  right : Inport
  left : Inport  Port=2
  Bus Selector : BusSelector  OutputSignals=MSG_Type,gripper,position,orientation (quat),MTM_time,Delay
  Bus Selector1 : BusSelector  OutputSignals=MSG_Type,gripper,position,orientation (quat)
  EN_fileSC : Constant  Value=0
  Gain : Gain
  Gain1 : Gain
  Left_MTM : slrtlib/Displays and Logging/Scope   scopeno=21  scopetype=Target  autostart=on  viewmode=Numerical  formatstr=scope_format_DaVinciMTML  grid=on  ylimits=[0,0]  nosamples=25  noprepostsamples=0  interleave=1  triggermode=FreeRun  triggersignal=1  trigsignalfromport=off  triggerlevel=0.0  triggerslope=Either  triggerscope=1  triggersample=0  filename=data.dat  mode=Lazy  writesize=512  autorestart=off  dynamicfilemode=off  maxwritefilesize=512*1024^2
  Mux : Mux  Inputs=5
  Mux1 : Mux  Inputs=2
  Mux2 : Mux
  Mux3 : Mux  Inputs=2
  Quaternion To Rotation : MATLAB Function  TreatAsAtomicUnit=on
  Quaternion To Rotation1 : MATLAB Function  TreatAsAtomicUnit=on
  R_to_axis_angle1 : MATLAB Function  TreatAsAtomicUnit=on
  R_to_axis_angle2 : MATLAB Function  TreatAsAtomicUnit=on
  Right_MTM : slrtlib/Displays and Logging/Scope   scopeno=19  scopetype=Host  autostart=on  viewmode=Numerical  formatstr=scope_format_DaVinciMTMR  grid=on  ylimits=[0,0]  nosamples=25  noprepostsamples=0  interleave=1  triggermode=FreeRun  triggersignal=1  trigsignalfromport=off  triggerlevel=0.0  triggerslope=Either  triggerscope=1  triggersample=0  filename=data.dat  mode=Lazy  writesize=512  autorestart=off  dynamicfilemode=off  maxwritefilesize=512*1024^2
  Terminator : Terminator
  to file : Subsystem
  wires:
  right/1 -> Bus Selector/1
  Quaternion To Rotation/1(R) -> R_to_axis_angle1/1(R)
  R_to_axis_angle1/1(n_vec) -> Mux1/1
  R_to_axis_angle1/2(theta) -> Mux1/2
  Bus Selector/1 -> Mux/1  "<MSG_Type>"
  Bus Selector/2 -> Mux/2  "<gripper>"
  Mux/1 -> Gain/1
  Bus Selector/4 -> Quaternion To Rotation/1(quat)  "<orientation (quat)>"
  Mux1/1 -> Mux/4
  Bus Selector/3 -> Mux/3  "<position>"
  Quaternion To Rotation1/1(R) -> R_to_axis_angle2/1(R)
  R_to_axis_angle2/1(n_vec) -> Mux3/1
  R_to_axis_angle2/2(theta) -> Mux3/2
  Bus Selector1/1 -> Mux2/1  "<MSG_Type>"
  Bus Selector1/2 -> Mux2/2  "<gripper>"
  Bus Selector1/4 -> Quaternion To Rotation1/1(quat)  "<orientation (quat)>"
  Mux3/1 -> Mux2/4
  Bus Selector1/3 -> Mux2/3  "<position>"
  Mux2/1 -> Gain1/1
  left/1 -> Bus Selector1/1
  Gain/1 -> Right_MTM/1, to file/1(right)
  Gain1/1 -> Left_MTM/1, to file/2(left)
  Bus Selector/5 -> Terminator/1  "<MTM_time>"
  Bus Selector/6 -> Mux/5  "<Delay>"
  EN_fileSC/1 -> to file/Enable

== system irep_force_control_simu/In-Vivo System/ATI FT Sensor ==
  ATI FT Sensor - 20001 : xpcrtudplib/Legacy UDP/Receive   ipAddress=0.0.0.0  ipPort=20001  width=48  vblLen=on  sampletime=2*dt
  Mux1 : Mux  Inputs=6
  Terminator1 : Terminator
  Unpack 2 : xpcobsoletelib/Utilities/Unpack   dimensions={1,1,1,1,1,1}  datatypes={'double' 'double' 'double' 'double' 'double' 'double'}  byteAlign=1
  Forces : Outport
  wires:
  ATI FT Sensor - 20001/1 -> Unpack 2/1
  ATI FT Sensor - 20001/2 -> Terminator1/1
  Unpack 2/2 -> Mux1/2  "Fy"
  Unpack 2/3 -> Mux1/3  "Fz"
  Unpack 2/4 -> Mux1/4  "Mx"
  Unpack 2/5 -> Mux1/5  "My"
  Unpack 2/6 -> Mux1/6  "Mz"
  Mux1/1 -> Forces/1
  Unpack 2/1 -> Mux1/1  "Fx"

== system irep_force_control_simu/In-Vivo System/CONTEC CARDS ==
  Level 1 : Subsystem
  Level 2 : Subsystem
  Level 3 : Subsystem
  Mux : Mux
  RZ : Subsystem
  Out1 : Outport
  wires:
  Level 1/1(Out1) -> Mux/1
  Level 2/1(Out1) -> Mux/2
  Level 3/1(Out1) -> Mux/3
  Mux/1 -> Out1/1
  RZ/1(Out1) -> Mux/4

== system irep_force_control_simu/In-Vivo System/Count to mm ==
  counts : Inport
  Bus Creator : Subsystem
  Subtract : Sum  Inputs=+-
  counter_offset : Constant  Value=counter_offset*ones(23,1)  SampleTime=dt
  counts  to mm : Gain  Gain=screw_pitch./(quadrature_mode*encoder_counts.*gear_ratio)  SampleTime=dt
  q_cur_system : Outport
  wires:
  Subtract/1 -> counts  to mm/1
  counter_offset/1 -> Subtract/2
  counts/1 -> Subtract/1
  Bus Creator/1(Out1) -> q_cur_system/1
  counts  to mm/1 -> Bus Creator/1(In1)

== system irep_force_control_simu/In-Vivo System/D/A ==
  In1 : Inport
  Bus Selector 1 : Subsystem
  Bus Selector 2 : Subsystem
  Bus Selector 3 : Subsystem
  Level 1 : Subsystem
  Level 2 : Subsystem
  Level 3 : Subsystem
  Parker Level : Subsystem
  wires:
  Bus Selector 1/1(Out1) -> Level 1/1(In1)
  Bus Selector 2/1(Out1) -> Level 2/1(In1)
  Bus Selector 3/1(Out1) -> Level 3/1(In1)
  In1/1 -> Bus Selector 2/1(In1), Bus Selector 1/1(In1), Bus Selector 3/1(In1), Parker Level/1(In1)

== system irep_force_control_simu/In-Vivo System/Digital_Inputs ==
  note: All the digital I/O input, when 0 meaning "enable" or "yes"
  note: Right foot switch
      | PCI-DAS1602/12
      | Digital Input
      | Slot: [2, 9]
      | Port B
      | Channel [2]
  note: Left foot swith
      | PCI-DAS1602/12
      | Digital Input
      | Slot: [2, 9]
      | Port B
      | Channel [1]
  note: Right Pot Front connect
      | PCI-DAS1602/12
      | Digital Input
      | Slot: [2, 9]
      | Port B
      | Channel [3]
  note: Right Pot Rear connect
      | PCI-DAS1602/12
      | Digital Input
      | Slot: [2, 9]
      | Port B
      | Channel [4]
  note: Left Pot Front connect
      | PCI-DAS1602/12
      | Digital Input
      | Slot: [2, 9]
      | Port B
      | Channel [5]
  note: Left Pot Rear connect
      | PCI-DAS1602/12
      | Digital Input
      | Slot: [2, 9]
      | Port B
      | Channel [6]
  Bus Creator1 : BusCreator  Inputs=2
  Bus Creator2 : BusCreator  Inputs=2
  Constant{,1..5} (6 alike) : Constant
  Mux : Mux  Inputs=2
  Mux1 : Mux  Inputs=2
  foot switches : Outport
  Pot_connect : Outport  Port=2
  wires:
  Constant1/1 -> Bus Creator1/2  "left foot switch"
  Constant/1 -> Bus Creator1/1  "right foot switch"
  Bus Creator1/1 -> foot switches/1
  Bus Creator2/1 -> Pot_connect/1
  Constant2/1 -> Mux/1
  Constant3/1 -> Mux/2
  Constant4/1 -> Mux1/1
  Constant5/1 -> Mux1/2
  Mux/1 -> Bus Creator2/1  "R_Pots_Connect"
  Mux1/1 -> Bus Creator2/2  "L_Pots_Connect"

== system irep_force_control_simu/In-Vivo System/Loadcells ==
  note: Measurement computing
      | PCI-DAS1602/12
      | range [+/- 10V]
      | Differential
      | Slot:[2, 12]
      | 8 channels
  Bus Creator : BusCreator  Inputs=2
  Constant{,1..7} (8 alike) : Constant  Value=0
  Force Bias : Constant  Value=LOADCELL_BIAS
  Gain : Gain  Gain=LOADCELL_GAIN  Multiplication=Matrix(K*u)
  Loadcell Backbone Mapping : Subsystem
  Manual LC Bias : Constant  Value=zeros(8,1)
  Mux : Mux  Inputs=8
  Sum : Sum  Inputs=|+-
  Sum1 : Sum  Inputs=|+-
  unbiased : Gain
  loadcell : Outport
  wires:
  Mux/1 -> Sum/1
  Sum/1 -> Gain/1
  Force Bias/1 -> Sum/2
  Bus Creator/1 -> loadcell/1  "force_sensing"
  Loadcell Backbone Mapping/1(tau backbones) -> Bus Creator/2  "tau_backbones"
  Sum1/1 -> unbiased/1
  Gain/1 -> Sum1/1
  Manual LC Bias/1 -> Sum1/2
  unbiased/1 -> Loadcell Backbone Mapping/1(loadcell reading), Bus Creator/1  "loadcell"
  Constant/1 -> Mux/1
  Constant1/1 -> Mux/2
  Constant2/1 -> Mux/3
  Constant3/1 -> Mux/4
  Constant4/1 -> Mux/5
  Constant5/1 -> Mux/6
  Constant6/1 -> Mux/7
  Constant7/1 -> Mux/8

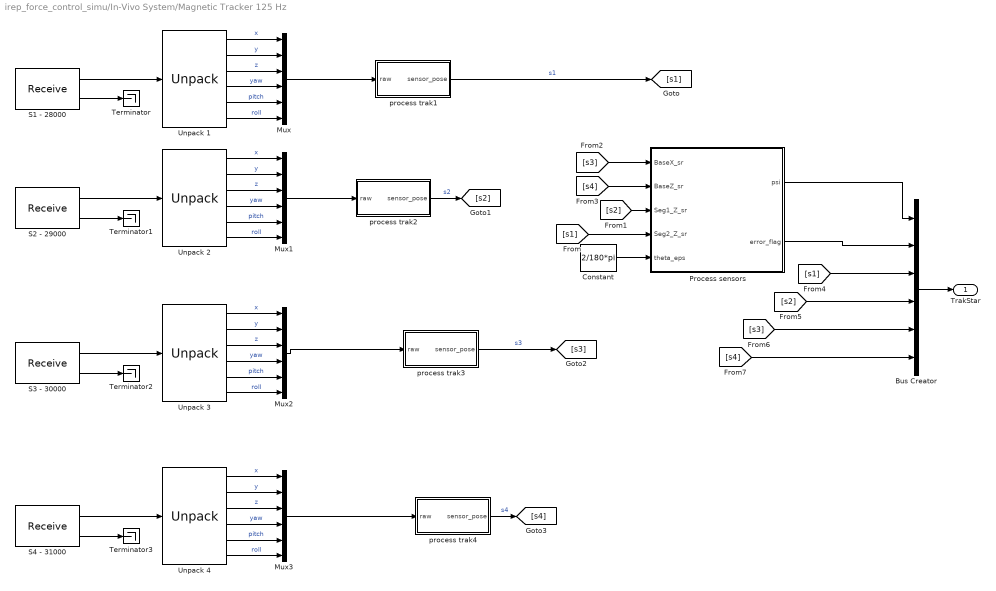
== system irep_force_control_simu/In-Vivo System/Magnetic Tracker 125 Hz ==
  Bus Creator : BusCreator  Inputs=6
  Constant : Constant  Value=2/180*pi
  Mux{,1..3} (4 alike) : Mux  Inputs=6
  Process sensors : MATLAB Function  TreatAsAtomicUnit=on
  S1 - 28000 : xpcrtudplib/Legacy UDP/Receive   ipAddress=0.0.0.0  ipPort=28000  width=48  vblLen=on  sampletime=dt_trakstar
  S2 - 29000 : xpcrtudplib/Legacy UDP/Receive   ipAddress=0.0.0.0  ipPort=29000  width=48  vblLen=on  sampletime=dt_trakstar
  S3 - 30000 : xpcrtudplib/Legacy UDP/Receive   ipAddress=0.0.0.0  ipPort=30000  width=48  vblLen=on  sampletime=dt_trakstar
  S4 - 31000 : xpcrtudplib/Legacy UDP/Receive   ipAddress=0.0.0.0  ipPort=31000  width=48  vblLen=on  sampletime=dt_trakstar
  Terminator{,1..3} (4 alike) : Terminator
  Unpack {1..4} (4 alike) : xpcobsoletelib/Utilities/Unpack   dimensions={1,1,1,1,1,1}  datatypes={'double' 'double' 'double' 'double' 'double' 'double'}  byteAlign=1
  process trak1 : Subsystem
  process trak2 : Subsystem
  process trak3 : Subsystem
  process trak4 : Subsystem
  TrakStar : Outport
  wires:
  S1 - 28000/1 -> Unpack 1/1
  S1 - 28000/2 -> Terminator/1
  Unpack 1/1 -> Mux/1  "x"
  Unpack 1/2 -> Mux/2  "y"
  Unpack 1/3 -> Mux/3  "z"
  Unpack 1/4 -> Mux/4  "yaw"
  Unpack 1/5 -> Mux/5  "pitch"
  Unpack 1/6 -> Mux/6  "roll"
  Mux/1 -> process trak1/1(raw)
  S2 - 29000/1 -> Unpack 2/1
  S2 - 29000/2 -> Terminator1/1
  Unpack 2/1 -> Mux1/1  "x"
  Unpack 2/2 -> Mux1/2  "y"
  Unpack 2/3 -> Mux1/3  "z"
  Unpack 2/4 -> Mux1/4  "yaw"
  Unpack 2/5 -> Mux1/5  "pitch"
  Unpack 2/6 -> Mux1/6  "roll"
  Mux1/1 -> process trak2/1(raw)
  Bus Creator/1 -> TrakStar/1
  S3 - 30000/1 -> Unpack 3/1
  S3 - 30000/2 -> Terminator2/1
  Unpack 3/1 -> Mux2/1  "x"
  Unpack 3/2 -> Mux2/2  "y"
  Unpack 3/3 -> Mux2/3  "z"
  Unpack 3/4 -> Mux2/4  "yaw"
  Unpack 3/5 -> Mux2/5  "pitch"
  Unpack 3/6 -> Mux2/6  "roll"
  Mux2/1 -> process trak3/1(raw)
  S4 - 31000/1 -> Unpack 4/1
  S4 - 31000/2 -> Terminator3/1
  Unpack 4/1 -> Mux3/1  "x"
  Unpack 4/2 -> Mux3/2  "y"
  Unpack 4/3 -> Mux3/3  "z"
  Unpack 4/4 -> Mux3/4  "yaw"
  Unpack 4/5 -> Mux3/5  "pitch"
  Unpack 4/6 -> Mux3/6  "roll"
  Mux3/1 -> process trak4/1(raw)
  Constant/1 -> Process sensors/5(theta_eps)
  Process sensors/1(psi) -> Bus Creator/1
  [s1] -> Process sensors/4(Seg2_Z_sr)
  process trak2/1(sensor_pose) -> [s2]  "s2"
  [s2] -> Process sensors/3(Seg1_Z_sr)
  process trak3/1(sensor_pose) -> [s3]  "s3"
  [s3] -> Process sensors/1(BaseX_sr)
  process trak4/1(sensor_pose) -> [s4]  "s4"
  [s4] -> Process sensors/2(BaseZ_sr)
  [s4] -> Bus Creator/6
  [s3] -> Bus Creator/5
  [s2] -> Bus Creator/4
  [s1] -> Bus Creator/3
  Process sensors/2(error_flag) -> Bus Creator/2
  process trak1/1(sensor_pose) -> [s1]  "s1"

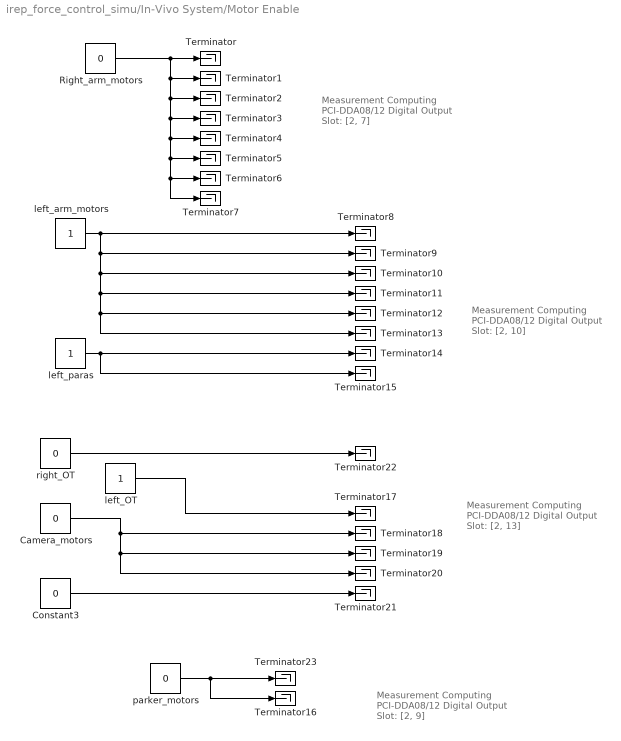
== system irep_force_control_simu/In-Vivo System/Motor Enable ==
  note: Measurement Computing
      | PCI-DDA08/12
      | Digital Output
      | Slot: [2, 7]
  note: Measurement Computing
      | PCI-DDA08/12
      | Digital Output
      | Slot: [2, 10]
  note: Measurement Computing
      | PCI-DDA08/12
      | Digital Output
      | Slot: [2, 13]
  note: Measurement Computing
      | PCI-DDA08/12
      | Digital Output
      | Slot: [2, 9]
  Camera_motors : Constant  Value=0
  Constant3 : Constant  Value=0
  Right_arm_motors : Constant  Value=0
  Terminator{,1..23} (24 alike) : Terminator
  left_OT : Constant
  left_arm_motors : Constant
  left_paras : Constant
  parker_motors : Constant  Value=0
  right_OT : Constant  Value=0
  wires:
  Right_arm_motors/1 -> Terminator7/1, Terminator6/1, Terminator5/1, Terminator4/1, Terminator3/1, Terminator2/1, Terminator1/1, Terminator/1
  left_arm_motors/1 -> Terminator13/1, Terminator12/1, Terminator11/1, Terminator10/1, Terminator9/1, Terminator8/1
  Camera_motors/1 -> Terminator20/1, Terminator19/1, Terminator18/1
  Constant3/1 -> Terminator21/1
  left_paras/1 -> Terminator15/1, Terminator14/1
  parker_motors/1 -> Terminator23/1, Terminator16/1
  right_OT/1 -> Terminator22/1
  left_OT/1 -> Terminator17/1

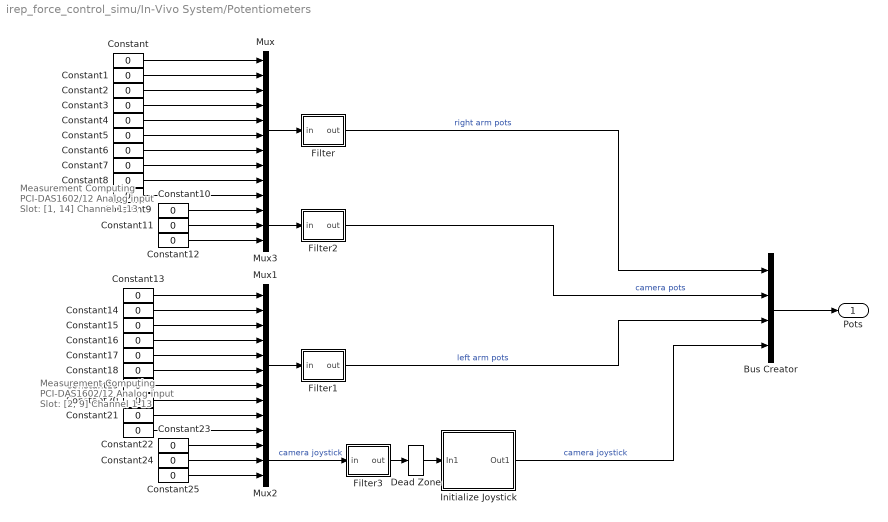
== system irep_force_control_simu/In-Vivo System/Potentiometers ==
  note: Measurement Computing
      | PCI-DAS1602/12
      | Analog input
      | Slot: [1, 14]
      | Channel 1-13
  note: Measurement Computing
      | PCI-DAS1602/12
      | Analog input
      | Slot: [2, 9]
      | Channel 1-13
  Bus Creator : BusCreator
  Constant{,1..25} (26 alike) : Constant  Value=0
  Dead Zone : DeadZone  LowerValue=2.5-0.4  UpperValue=2.5+0.4  SaturateOnIntegerOverflow=on
  Filter : Subsystem
  Filter1 : Subsystem
  Filter2 : Subsystem
  Filter3 : Subsystem
  Initialize Joystick : Subsystem
  Mux : Mux  Inputs=10
  Mux1 : Mux  Inputs=10
  Mux2 : Mux  Inputs=3
  Mux3 : Mux  Inputs=3
  Pots : Outport
  wires:
  Bus Creator/1 -> Pots/1
  Mux/1 -> Filter/1(in)
  Filter1/1(out) -> Bus Creator/3  "left arm pots"
  Mux1/1 -> Filter1/1(in)
  Mux2/1 -> Filter3/1(in)  "camera joystick"
  Initialize Joystick/1(Out1) -> Bus Creator/4  "camera joystick"
  Filter/1(out) -> Bus Creator/1  "right arm pots"
  Mux3/1 -> Filter2/1(in)
  Filter2/1(out) -> Bus Creator/2  "camera pots"
  Dead Zone/1 -> Initialize Joystick/1(In1)
  Filter3/1(out) -> Dead Zone/1
  Constant/1 -> Mux/1
  Constant1/1 -> Mux/2
  Constant2/1 -> Mux/3
  Constant3/1 -> Mux/4
  Constant4/1 -> Mux/5
  Constant5/1 -> Mux/6
  Constant6/1 -> Mux/7
  Constant7/1 -> Mux/8
  Constant8/1 -> Mux/9
  Constant9/1 -> Mux/10
  Constant10/1 -> Mux3/1
  Constant11/1 -> Mux3/2
  Constant12/1 -> Mux3/3
  Constant13/1 -> Mux1/1
  Constant14/1 -> Mux1/2
  Constant15/1 -> Mux1/3
  Constant16/1 -> Mux1/4
  Constant17/1 -> Mux1/5
  Constant18/1 -> Mux1/6
  Constant19/1 -> Mux1/7
  Constant20/1 -> Mux1/8
  Constant21/1 -> Mux1/9
  Constant22/1 -> Mux1/10
  Constant23/1 -> Mux2/1
  Constant24/1 -> Mux2/2
  Constant25/1 -> Mux2/3

== system irep_force_control_simu/In-Vivo System/motor simulation ==
  note: Here the simulation neglects the dynamics
      | assuming the q_des will be the q_cur in next time step
  u : Inport
  Bus Creator : Subsystem
  motor simu : Subsystem
  q_des to q_cur mapping : Subsystem
  u mapping : Subsystem
  q_cur_system : Outport
  wires:
  Bus Creator/1(Out1) -> q_cur_system/1
  u/1 -> u mapping/1(u in)
  q_des to q_cur mapping/1(q cur out) -> Bus Creator/1(In1)
  motor simu/1(q cur) -> q_des to q_cur mapping/1(q cur in)
  u mapping/1(u out) -> motor simu/1(u)

== system irep_force_control_simu/Joint Level PID Control in mm/Bus Creator ==
  In1 : Inport
  Bus Creator : BusCreator  Inputs=23
  Demux : Demux  Outputs=23
  Out1 : Outport
  wires:
  Demux/1 -> Bus Creator/1  "Righ arm - Overall Translational Movement"
  Demux/2 -> Bus Creator/2  "Right arm - Parallelogram Insert"
  Demux/3 -> Bus Creator/3  "Right arm - Parallelogram Deploy"
  Demux/4 -> Bus Creator/4  "Right arm - Proximal Segment X"
  Demux/5 -> Bus Creator/5  "Right arm - Proximal Segment Y"
  Demux/6 -> Bus Creator/6  "Right arm - Distal Segment X"
  Demux/7 -> Bus Creator/7  "Right arm - Distal Segment Y"
  Demux/8 -> Bus Creator/8  "Right arm - Wrist Joint"
  Demux/9 -> Bus Creator/9  "Right arm - Gripper Joint"
  Demux/10 -> Bus Creator/10  "Left arm - Overall Translational Movement"
  Demux/11 -> Bus Creator/11  "Left arm - Parallelogram Insert"
  Demux/12 -> Bus Creator/12  "Left arm - Parallelogram Deploy"
  Demux/13 -> Bus Creator/13  "Left arm - Proximal Segment X"
  Demux/14 -> Bus Creator/14  "Left arm - Proximal Segment Y"
  Demux/15 -> Bus Creator/15  "Left arm - Distal Segment X"
  Demux/16 -> Bus Creator/16  "Left arm - Distal Segment Y"
  Demux/17 -> Bus Creator/17  "Left arm - Wrist Joint"
  Demux/18 -> Bus Creator/18  "Left arm - Gripper Joint"
  Demux/19 -> Bus Creator/19  "Camera shell open"
  Demux/20 -> Bus Creator/20  "Camera Pan"
  Demux/21 -> Bus Creator/21  "Camera Tilt"
  Bus Creator/1 -> Out1/1
  In1/1 -> Demux/1
  Demux/22 -> Bus Creator/22  "Parker insertion stage"
  Demux/23 -> Bus Creator/23  "Parker rotary stage"

== system irep_force_control_simu/Joint Level PID Control in mm/Bus selector ==
  sensors : Inport
  Camera selector : Subsystem
  Left arm selector : Subsystem
  Mux : Mux
  RZ : Subsystem
  Right arm  selector : Subsystem
  Out1 : Outport
  wires:
  Left arm selector/1(Out1) -> Mux/2
  Right arm  selector/1(Out1) -> Mux/1
  Camera selector/1(Out1) -> Mux/3
  Mux/1 -> Out1/1
  sensors/1 -> Left arm selector/1(In1), Right arm  selector/1(In1), Camera selector/1(In1), RZ/1(In1)
  RZ/1(Out1) -> Mux/4
